simulink model "update"  (R2014b)
settings: Solver=ode45  StartTime=0.0  StopTime=10.0  RelTol=1e-3
values from neighbouring files (symbols this model uses):
  fluid =     [fpropsR134a.mat]    (also in run.m = rmfield(fluid,'name'))
undefined symbols (not defined in the file or in its folder): stateA
settings Model: Creator=emiller  LastModifiedBy=emiller

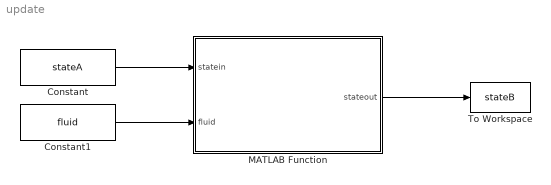
== system update ==
  Constant : Constant  Value=stateA  OutDataTypeStr=Bus: stateAbus
  Constant1 : Constant  Value=fluid  OutDataTypeStr=Bus: fluidBus
  MATLAB Function : MATLAB Function  TreatAsAtomicUnit=on
  To Workspace : ToWorkspace  VariableName=stateB  SaveFormat=Timeseries  SampleTime=-1
  wires:
  Constant/1 -> MATLAB Function/1(statein)
  MATLAB Function/1(stateout) -> To Workspace/1
  Constant1/1 -> MATLAB Function/2(fluid)

== matlab function update/MATLAB Function ==
  data: statein input Bus: stateAbus; stateout output Bus: stateAbus; fluid input Bus: fluidBus
function stateout = update(statein,fluid)
%#codegen
stateout=statein;
% fluid=stateout.fluid;
%Check Dimensions
if stateout.dimensions == 1
    h=stateout.enthalpy./stateout.mass;
else
    h=stateout.specificenthalpy;
end
%Check for Phase Change Fluid
if stateout.phases == 2
    p=stateout.pressure;
    stateout.temperature=interp2DUG(fluid.PP,fluid.HH,fluid.T_P_H,p,h);
    stateout.density=interp2DUG(fluid.PP,fluid.HH,fluid.D_P_H,p,h);
    stateout.quality=interp2DUG(fluid.PP,fluid.HH,fluid.Q_P_H,p,h);
elseif stateout.phases == 1
    stateout.temperature=interp1DUG(fluid.HH,fluid.T_H,h);
    stateout.density=interp1DUG(fluid.HH,fluid.D_H,h);
else
    error('unable to read fluid type in Props')
end
